simulink library "cda"  (Simulink 8.1)
settings: Solver=ode1  StartTime=0.0  StopTime=Inf  FixedStep=0.001  RelTol=1e-3
PostLoadFcn:
  | , if any(exist('dsrtsu_mdlpostloadfcn', 'file') == [2, 3, 6]), try dsrtsu_mdlpostloadfcn('Execute', bdroot); catch fprintf('Error in PostLoadFcn (dsrtsu_mdlpostloadfcn) for model "%s":\n %s\n', bdroot, lasterr); end, end,
undefined symbols (not defined in the file or in its folder): C_TICK_TIME_S, ENUM_AEBSTATE_AUTOBRAKING, FALSE, KJUD_ACCDeactVehSpeed_kph, KJUD_ACCOverrideTimer_s, KJUD_ACCVehAssignMaintTime_ms, TRUE, ZERO_INT
libraries: cva x1, gbp x1
settings Model: DSRTSU_INTERNAL_RTI_VER=450  DSRTSU_INTERNAL_RTI_TYPE=rti1401  RTICANMMDATA=struct('GeneralSetupData',struct('modelroot','D:\ELN150201_TAIWAN\trunk\AdasDragon\software\sw_development\arch\app\jud','generalsettings',struct('filesettings',struct('destfolder',struct('Name','RTICANMM_FILES','Check',1),'buildfolder',struct('Name','.','Check',1),'AbsDestfolder',struct('Name','D:\ELN150201_TAIWAN\trunk\AdasDragon\software\sw_development\arch\app\jud\RTICANMM_FILES'),'AbsBuildfolder',struct('Name','D:\ELN150201_TAIWAN\trunk\AdasDragon\software\sw_development\arch\app\jud'))),'options',struct('addpaths',1,'rmpaths',1,'addtrcexclusion',logical(1),'cannavigator',struct('checkmonitoring',0),'show_usrtrc',0,'use_usrtrc',0),'advanced',struct('options',[1 1 1 1 1 1 1 1 1 1 1 1 1 1 1 1 1 1 1 1 1 1 1 1 1 1 1 1 1 1 1 1 1 1 1 1 1 1 1 1 1 1 1 1 1 1 1 1 1 1 1 1 1 1 1 1 1 1 1 1 1 1 1 1 1 1 1 1 1 1 1 1 1 1 1 1 1 1 1 1 1 1 1 1 1 1 1 1 1 1 1 1 1 1 1 1 1 1 1 1]),'MPSetup',{{}},'modelname','cda','block','cda'))  DSRTSU_INTERNAL_RTIFPGA=40  Creator=AT015411  LastModifiedBy=AT015555

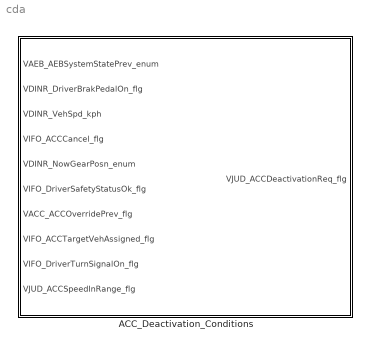
== system cda ==
  ACC_Deactivation_Conditions : Subsystem

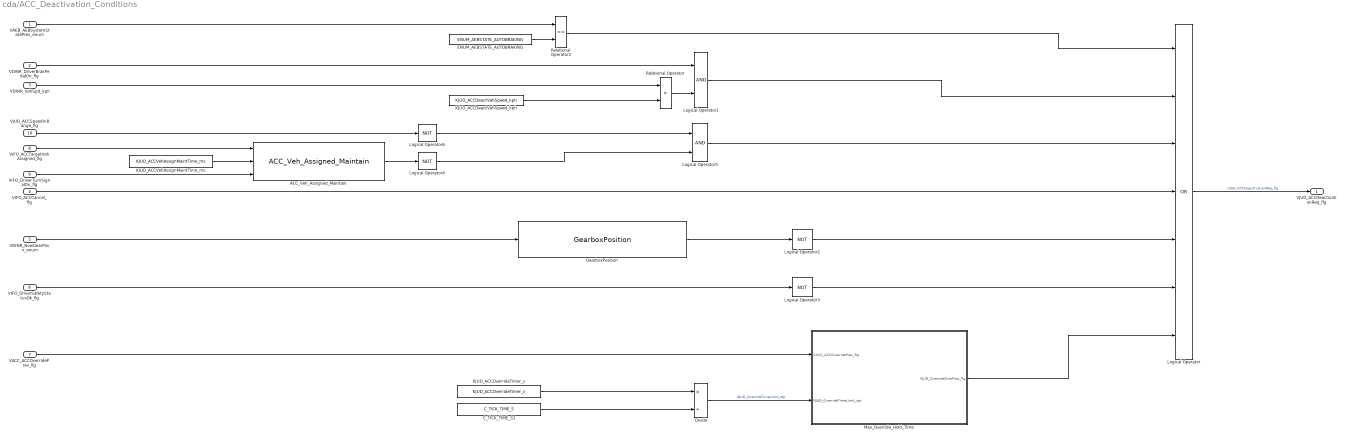
== system cda/ACC_Deactivation_Conditions ==
  VAEB_AEBSystemStatePrev_enum : Inport
  VDINR_DriverBrakPedalOn_flg : Inport  Port=2
  VDINR_VehSpd_kph : Inport  Port=3
  VIFO_ACCCancel_flg : Inport  Port=4
  VDINR_NowGearPosn_enum : Inport  Port=5
  VIFO_DriverSafetyStatusOk_flg : Inport  Port=6
  VACC_ACCOverridePrev_flg : Inport  Port=7
  VIFO_ACCTargetVehAssigned_flg : Inport  Port=8
  VIFO_DriverTurnSignalOn_flg : Inport  Port=9
  VJUD_ACCSpeedInRange_flg : Inport  Port=10
  ACC_Veh_Assigned_Maintain : cva/ACC_Veh_Assigned_Maintain
  C_TICK_TIME_S2 : Constant  Value=C_TICK_TIME_S  OutDataTypeStr=single
  Divide : Product  Inputs=*/
  ENUM_AEBSTATE_AUTOBRAKING : Constant  Value=ENUM_AEBSTATE_AUTOBRAKING
  GearboxPosition : gbp/GearboxPosition
  KJUD_ACCDeactVehSpeed_kph : Constant  Value=KJUD_ACCDeactVehSpeed_kph
  KJUD_ACCOverrideTimer_s : Constant  Value=KJUD_ACCOverrideTimer_s  OutDataTypeStr=single
  KJUD_ACCVehAssignMaintTime_ms : Constant  Value=KJUD_ACCVehAssignMaintTime_ms
  Logical Operator : Logic  Operator=OR  Inputs=7  AllPortsSameDT=off  OutDataTypeStr=boolean
  Logical Operator1 : Logic  AllPortsSameDT=off  OutDataTypeStr=boolean
  Logical Operator2 : Logic  Operator=NOT  Inputs=5  AllPortsSameDT=off  OutDataTypeStr=boolean
  Logical Operator3 : Logic  Operator=NOT  Inputs=5  AllPortsSameDT=off  OutDataTypeStr=boolean
  Logical Operator4 : Logic  Operator=NOT  AllPortsSameDT=off  OutDataTypeStr=boolean
  Logical Operator5 : Logic  AllPortsSameDT=off  OutDataTypeStr=boolean
  Logical Operator6 : Logic  Operator=NOT  AllPortsSameDT=off  OutDataTypeStr=boolean
  Max_Override_Hold_Time : Stateflow chart  TreatAsAtomicUnit=on
  Relational Operator : RelationalOperator  Operator=>  OutDataTypeStr=boolean
  Relational Operator2 : RelationalOperator  Operator===  OutDataTypeStr=boolean
  VJUD_ACCDeactivationReq_flg : Outport
  wires:
  Logical Operator/1 -> VJUD_ACCDeactivationReq_flg/1  "VJUD_ACCDeactivationReq_flg"
  Relational Operator/1 -> Logical Operator1/2
  VDINR_DriverBrakPedalOn_flg/1 -> Logical Operator1/1
  VDINR_VehSpd_kph/1 -> Relational Operator/1
  VAEB_AEBSystemStatePrev_enum/1 -> Relational Operator2/1
  Logical Operator1/1 -> Logical Operator/2
  VIFO_ACCCancel_flg/1 -> Logical Operator/4
  VACC_ACCOverridePrev_flg/1 -> Max_Override_Hold_Time/1(VACC_ACCOverridePrev_flg)
  KJUD_ACCOverrideTimer_s/1 -> Divide/1
  Divide/1 -> Max_Override_Hold_Time/2(NJUD_OverrideTimeLimit_stp)  "NJUD_OverrideTimeLimit_stp"
  C_TICK_TIME_S2/1 -> Divide/2
  Max_Override_Hold_Time/1(VJUD_OverrideOverflow_flg) -> Logical Operator/7
  VDINR_NowGearPosn_enum/1 -> GearboxPosition/1
  Logical Operator2/1 -> Logical Operator/5
  KJUD_ACCDeactVehSpeed_kph/1 -> Relational Operator/2
  GearboxPosition/1 -> Logical Operator2/1
  VIFO_DriverSafetyStatusOk_flg/1 -> Logical Operator3/1
  Logical Operator3/1 -> Logical Operator/6
  Relational Operator2/1 -> Logical Operator/1
  ENUM_AEBSTATE_AUTOBRAKING/1 -> Relational Operator2/2
  VIFO_ACCTargetVehAssigned_flg/1 -> ACC_Veh_Assigned_Maintain/1
  Logical Operator4/1 -> Logical Operator5/2
  Logical Operator5/1 -> Logical Operator/3
  ACC_Veh_Assigned_Maintain/1 -> Logical Operator4/1
  KJUD_ACCVehAssignMaintTime_ms/1 -> ACC_Veh_Assigned_Maintain/2
  VIFO_DriverTurnSignalOn_flg/1 -> ACC_Veh_Assigned_Maintain/3
  VJUD_ACCSpeedInRange_flg/1 -> Logical Operator6/1
  Logical Operator6/1 -> Logical Operator5/1

== stateflow chart ACC_Deactivation_Conditions/Max_Override_Hold_Time ==
  state INITIAL
    en:
    VJUD_OverrideOverflow_flg =FALSE;
  state OVERRIDE
    en:
    NJUD_OverrideTimeLocal_stp = ZERO_INT;
    du:
    NJUD_OverrideTimeLocal_stp = NJUD_OverrideTimeLocal_stp+1;
  state OVERFLOW
    en:
    VJUD_OverrideOverflow_flg =TRUE;
  (default) -> INITIAL
  OVERRIDE -> OVERFLOW [order 1] : [NJUD_OverrideTimeLocal_stp>NJUD_OverrideTimeLimit_stp]
  INITIAL -> OVERRIDE : [VACC_ACCOverridePrev_flg==TRUE]
  OVERRIDE -> INITIAL [order 2] : [VACC_ACCOverridePrev_flg==FALSE]
  OVERFLOW -> INITIAL
  data: VACC_ACCOverridePrev_flg input double; NJUD_OverrideTimeLimit_stp input double; VJUD_OverrideOverflow_flg output single; FALSE parameter boolean; TRUE parameter boolean; NJUD_OverrideTimeLocal_stp local single; ZERO_INT parameter uint8
